simulink model "H_bot_model_PWM"  (R2023a)
settings: Solver=VariableStepAuto  StartTime=0.0  StopTime=1  RelTol=1e-3
undefined symbols (not defined in the file): A, B, C, D, theta_to_xy
settings Model: Creator=trent  LastModifiedBy=andre
settings OptimizationCC: ReuseModelBlockBuffer=off
settings DebuggingCC: UnconnectedInputMsg=warning  UnconnectedOutputMsg=warning  UnconnectedLineMsg=warning
settings ModelReferenceCC: EnableRefExpFcnMdlSchedulingChecks=on
settings RTWCC: DLArmComputeVersion=19.05

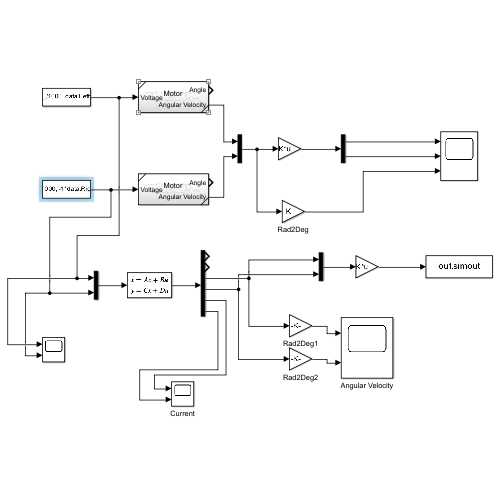
[thumbnail: Simulink's stored preview of the top-level diagram]
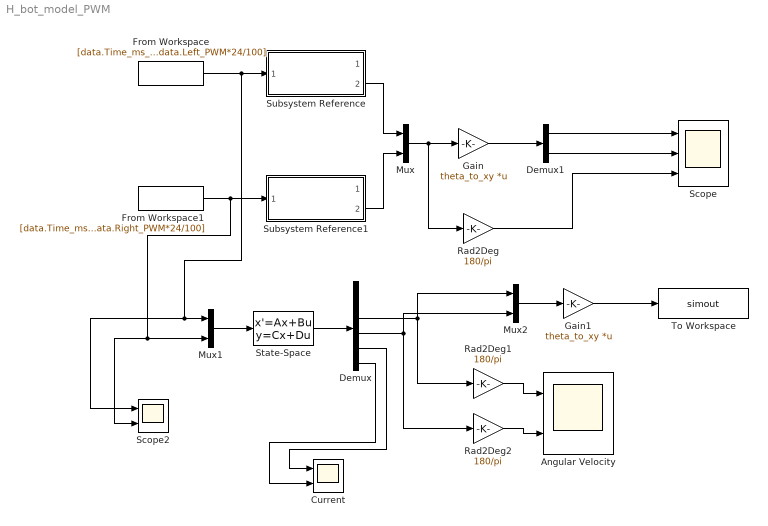
== system H_bot_model_PWM ==
  Angular Velocity : Scope  NumInputPorts=2
  Current : Scope  NumInputPorts=2
  Demux : Demux  Outputs=6
  Demux1 : Demux  Outputs=2
  From Workspace : FromWorkspace  VariableName=[data.Time_ms_/1000, data.Left_PWM*24/100]
  From Workspace1 : FromWorkspace  VariableName=[data.Time_ms_/1000, -1*data.Right_PWM*24/100]
  Gain : Gain  Gain=theta_to_xy  Multiplication=Matrix(K*u)
  Gain1 : Gain  Gain=theta_to_xy  Multiplication=Matrix(K*u)
  Mux : Mux  Inputs=2
  Mux1 : Mux  Inputs=2
  Mux2 : Mux  Inputs=2
  Rad2Deg : Gain  Gain=180/pi
  Rad2Deg1 : Gain  Gain=180/pi
  Rad2Deg2 : Gain  Gain=180/pi
  Scope : Scope  NumInputPorts=3
  Scope2 : Scope  NumInputPorts=2
  State-Space : StateSpace  A=A  B=B  C=[C; zeros(4,2) eye(4)]  D=[D; zeros(4,2)]  InitialCondition=[0;0;0;0;0;0];
  Subsystem Reference : Subsystem  ReferencedSubsystem=Motor
  Subsystem Reference1 : Subsystem  ReferencedSubsystem=Motor
  To Workspace : ToWorkspace  VariableName=simout  SaveFormat=Timeseries  SampleTime=-1
  wires:
  Mux/1 -> Gain/1, Rad2Deg/1
  Gain/1 -> Demux1/1
  Rad2Deg/1 -> Scope/3
  Demux1/2 -> Scope/2
  Demux1/1 -> Scope/1
  From Workspace/1 -> Mux1/1, Scope2/1, Subsystem Reference/1
  From Workspace1/1 -> Mux1/2, Scope2/2, Subsystem Reference1/1
  Subsystem Reference/2 -> Mux/1
  Subsystem Reference1/2 -> Mux/2
  Mux1/1 -> State-Space/1
  State-Space/1 -> Demux/1
  Demux/3 -> Mux2/1, Rad2Deg1/1
  Demux/4 -> Rad2Deg2/1, Mux2/2
  Mux2/1 -> Gain1/1
  Gain1/1 -> To Workspace/1
  Rad2Deg1/1 -> Angular Velocity/1
  Rad2Deg2/1 -> Angular Velocity/2
  Demux/5 -> Current/1
  Demux/6 -> Current/2
